simulink model "p2Sim"  (R2019a)
settings: Solver=ode4  StartTime=0.0  StopTime=10.0  FixedStep=0.001  RelTol=1e-3
undefined symbols (not defined in the file): controller, Discrete, dt, filter_R, plant_tf, sensor_tf, Time
libraries: ctrlSharedLib x1
settings Model: Creator=crs20  LastModifiedBy=crs20

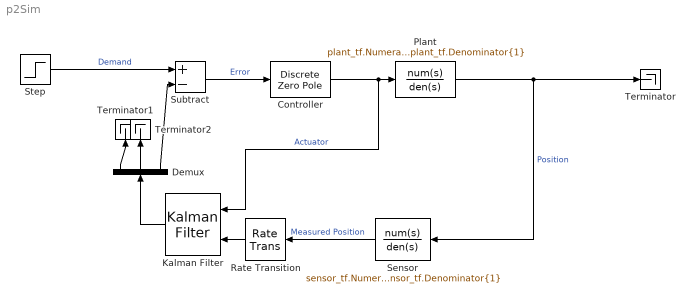
== system p2Sim ==
  Controller : DiscreteZeroPole  Zeros=controller.z{1}  Poles=controller.p{1}  Gain=controller.k  SampleTime=dt
  Demux : Demux  Outputs=3
  Kalman Filter : ctrlSharedLib/Kalman Filter  TimeDomain=Discrete-Time  UseCurrentEstimator=on  ModelSource=LTI State-Space Variable  ModelSourceVariable=filter_ss  A=0.95  B=1  C=1  D=0  NumberOfStates=1  NumberOfInputs=1  NumberOfOutputs=1  InitialEstimateSource=Dialog  X0=0  P0=10  UseK=off  UseGH=off  NumberOfProcessNoiseInputs=1  G=1  TimeInvariantG=on  H=0  TimeInvariantH=on  Q=filter_Q  TimeInvariantQ=on  R=filter_R  TimeInvariantR=on  N=0  TimeInvariantN=on  AddInputPort=on  AddEnablePort=off  OutputEstimatedY=off  OutputP=off  Ts=-1
      settings: SourceProductBaseCode=CT
  Plant : TransferFcn  Numerator=plant_tf.Numerator{1}  Denominator=plant_tf.Denominator{1}
  Rate Transition : RateTransition
  Sensor : TransferFcn  Numerator=sensor_tf.Numerator{1}  Denominator=sensor_tf.Denominator{1}
  Step : Step  Time=0  SampleTime=0
  Subtract : Sum  Inputs=+-
  Terminator : Terminator
  Terminator1 : Terminator
  Terminator2 : Terminator
  wires:
  Step/1 -> Subtract/1  "Demand"
  Plant/1 -> Sensor/1, Terminator/1  "Position"
  Subtract/1 -> Controller/1  "Error"
  Controller/1 -> Kalman Filter/1, Plant/1  "Actuator"
  Sensor/1 -> Rate Transition/1  "Measured Position"
  Kalman Filter/1 -> Demux/1
  Demux/3 -> Subtract/2
  Demux/1 -> Terminator1/1
  Demux/2 -> Terminator2/1
  Rate Transition/1 -> Kalman Filter/2
